simulink model "regulator_LQG_discrete_Ueq"  (R2022a)
settings: Solver=ode45  StartTime=0.0  StopTime=30  RelTol=1e-3  EnableMultiTasking=on
values from neighbouring files (symbols this model uses):
  Ad = dis_sys.A    [DC_motor.m]
  B_noise1 = [Bd Bw]    [DC_motor.m]
  Bw = [-0.0085 -0.0006 ... (first row only)    [DC_motor.m]
  Cd = dis_sys.C    [DC_motor.m]
  D_noise1 = [Dd Dd Dd]    [DC_motor.m]
  sat_max = Vmax    (= 12)    [DC_motor.m]
  sat_min = Vmin    (= 0)    [DC_motor.m]
  Ts = 1e-3    (= 0.001)    [DC_motor.m]
  W = [1 ... (first row only)    [DC_motor.m]
  x0 = [I0 n0]'    [DC_motor.m]
undefined symbols (not defined in the file or in its folder): Kdlqr
settings Model: Creator=Administrator  LastModifiedBy=jj
settings SolverCC: AlgebraicLoopSolver=TrustRegion
settings DataIOCC: LimitDataPoints=on  SaveFormat=Array  SignalLoggingSaveFormat=ModelDataLogs  ReturnWorkspaceOutputs=off
settings OptimizationCC: ExpressionDepthLimit=2147483647  InitFltsAndDblsToZero=on  LifeSpan=inf
settings DebuggingCC: UnderspecifiedInitializationDetection=Classic  MergeDetectMultiDrivingBlocksExec=none  SolverPrmCheckMsg=warning  FcnCallInpInsideContextMsg=warning  UnconnectedInputMsg=warning  UnconnectedOutputMsg=warning  UnconnectedLineMsg=warning  StateNameClashWarn=warning  SFUnexpectedBacktrackingDiag=warning  SFNoUnconditionalDefaultTransitionDiag=warning  SFExecutionAtInitializationDiag=none  SFMachineParentedDataDiag=warning  ArithmeticOperatorsInVariantConditions=warning
settings HardwareCC: ProdBitPerPointer=32  ProdBitPerSizeT=32  ProdBitPerPtrDiffT=32  ProdLargestAtomicFloat=None  ProdIntDivRoundTo=Undefined  ProdEndianess=Unspecified  ProdWordSize=32  ProdHWDeviceType=32-bit Generic
settings ModelReferenceCC: PropagateSignalLabelsOutOfModel=off
settings SFSimCC: SimUseLocalCustomCode=off  CustomCodeUndefinedFunction=UseInterfaceOnly
settings RTWCC: RTWUseLocalCustomCode=off
settings CodeAppCC: StateflowObjectComments=on
settings GRTTargetCC: TargetLangStandard=C89/C90 (ANSI)  CombineOutputUpdateFcns=off  GRTInterface=on
settings ConfigComp: CovMetricSettings=dw  CovSaveCumulativeToWorkspaceVar=on  CovSaveSingleToWorkspaceVar=on  CovExternalEMLEnable=off  CovSFcnEnable=off

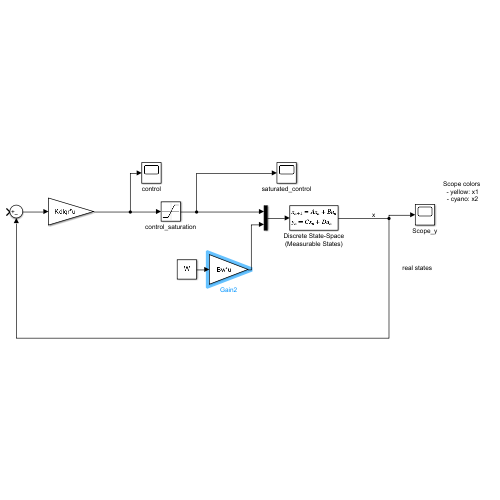
[thumbnail: Simulink's stored preview of the top-level diagram]
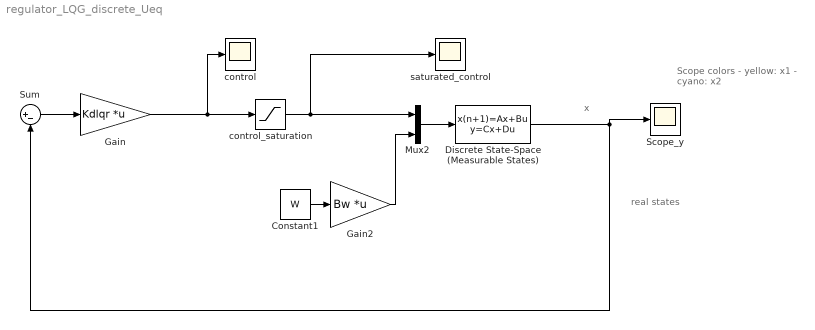
== system regulator_LQG_discrete_Ueq ==
  note: real states
  note: x
  note: Scope colors
      | - yellow: x1
      | - cyano: x2
  Constant1 : Constant  Value=W  SampleTime=Ts
  "Discrete State-Space (Measurable States) " : DiscreteStateSpace  A=Ad  B=B_noise1  C=Cd  D=D_noise1  InitialCondition=x0  SampleTime=Ts
  Gain : Gain  Gain=Kdlqr  Multiplication=Matrix(K*u)
  Gain2 : Gain  Gain=Bw  Multiplication=Matrix(K*u)
  Mux2 : Mux  Inputs=2
  Scope_y : Scope
  Sum : Sum  Inputs=|+-
  control : Scope
  control_saturation : Saturate  UpperLimit=sat_max  LowerLimit=sat_min
  saturated_control : Scope
  wires:
  Sum/1 -> Gain/1
  "Discrete State-Space (Measurable States) "/1 -> Scope_y/1, Sum/2
  control_saturation/1 -> Mux2/1, saturated_control/1
  Mux2/1 -> "Discrete State-Space (Measurable States) "/1
  Gain/1 -> control/1, control_saturation/1
  Constant1/1 -> Gain2/1
  Gain2/1 -> Mux2/2
